simulink model "autopilot3d"  (R2017a)
settings: Solver=VariableStepAuto  StartTime=0.0  StopTime=300  RelTol=1e-3
values from neighbouring files (symbols this model uses):
  A = [-0.322     0.052   0.028   -1.12   0.002 ... (first row only)    [run_task_3e.m]
  A_kal = A(1:4, 1:4)    [run_task_3e.m]
  B = [0; 0; 0; 0; 10]    [run_task_3e.m]
  B_kal = A(1:4,5)    [run_task_3e.m]
  C = [0 0 0 1 0 ... (first row only)    [run_task_3e.m]
  C_kal = [0 0 0 1 ... (first row only)    [run_task_3e.m]
  d = 2*deg2rad    (= 0.0349065850399)    [run_task_3e.m]
  D = zeros(4, 1)    [run_task_3e.m]
  g = 9.81    [run_task_3e.m]
  k_d_phi = (2*zeta_phi*w_n_phi-a_1)/a_2    [run_task_3e.m]
  k_i_x = 0.195    [run_task_3e.m]
  k_p_phi = -5/3    (= -1.66666666667)    [run_task_3e.m]
  k_p_x = 2*zeta_X*w_n_x*V_g/g    [run_task_3e.m]
  large_step = 30    [run_task_3e.m]
  P = [1 0 0 0 ... (first row only)    [run_task_3e.m]
  Q = [1 0 0 0 ... (first row only)    [run_task_3e.m]
  R = [r_noise_var 0 0 ... (first row only)    [run_task_3e.m]
  step_size = 0.001    [run_task_3e.m]
  V_g = 637/3.6    (= 176.944444444)    [run_task_3e.m]
  x_hat = x_hat_init    [run_task_3e.m]
libraries: simulink_extras x3
settings Model: Creator=rokru  LastModifiedBy=emilal

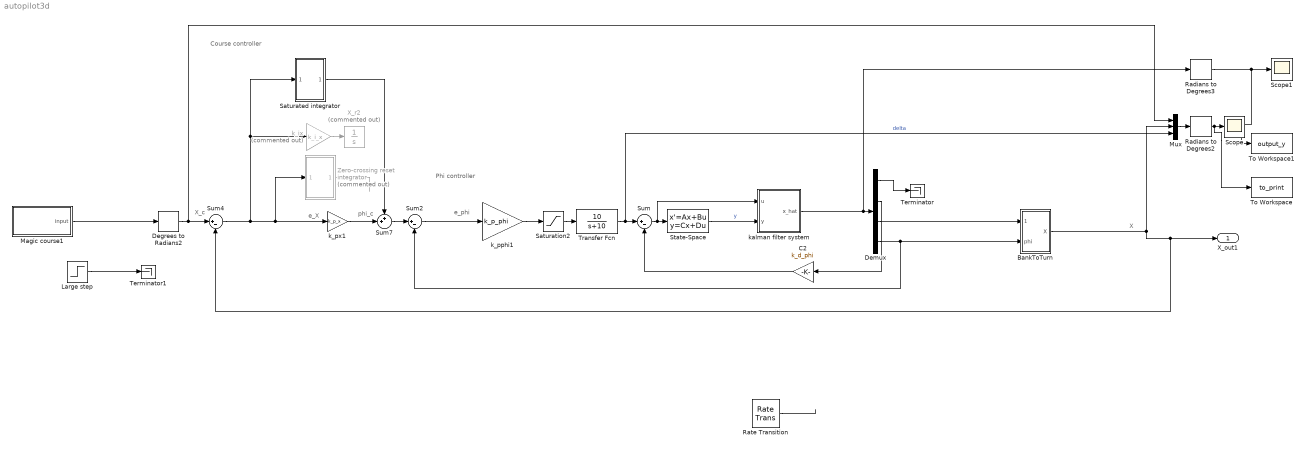
== system autopilot3d ==
  note: X
  note: X_c
  note: phi_c
  note: Course controller
  note: e_X
  note: Phi controller
  note: e_phi
  BankToTurn : Subsystem
  C2 : Gain  Gain=k_d_phi
  Degrees to Radians2 : simulink_extras/Transformations/Degrees to Radians
  Demux : Demux
  Large step : Step  Time=50  After=large_step  SampleTime=0
  Magic course1 : Subsystem
  Mux : Mux  Inputs=3
  Radians to Degrees2 : simulink_extras/Transformations/Radians to Degrees
  Radians to Degrees3 : simulink_extras/Transformations/Radians to Degrees
  Rate Transition : RateTransition
  Saturated integrator : Subsystem
  Saturation2 : Saturate  UpperLimit=25*deg2rad  LowerLimit=-25*deg2rad
  Scope : Scope
  Scope1 : Scope
  State-Space : StateSpace  A=A  B=B  C=C  D=D  X0=0
  Sum : Sum  Inputs=|+-
  Sum2 : Sum  Inputs=|+-
  Sum4 : Sum  Inputs=|+-
  Sum7 : Sum  Inputs=++|
  Terminator : Terminator
  Terminator1 : Terminator
  To Workspace : ToWorkspace  VariableName=to_print  SaveFormat=Timeseries  SampleTime=-1
  To Workspace1 : ToWorkspace  VariableName=output_y  SaveFormat=Timeseries  SampleTime=-1
  Transfer Fcn : TransferFcn  Numerator=[10]  Denominator=[1 10]
  X_r2 : Integrator  Commented=on
  "Zero-crossing reset integrator " : Subsystem  Commented=on
  k_ix : Gain  Commented=on  Gain=k_i_x
  k_pphi1 : Gain  Gain=k_p_phi
  k_px1 : Gain  Gain=k_p_x
  kalman filter system : Subsystem
  X_out1 : Outport
  wires:
  k_px1/1 -> Sum7/2
  Sum4/1 -> Saturated integrator/1(In1), k_ix/1, "Zero-crossing reset integrator "/1(In1), k_px1/1
  C2/1 -> Sum/2
  Saturation2/1 -> Transfer Fcn/1
  Mux/1 -> Radians to Degrees2/1
  Demux/2 -> C2/1
  Demux/4 -> Sum2/2, BankToTurn/2(phi)
  Sum/1 -> kalman filter system/1(u), State-Space/1
  k_pphi1/1 -> Saturation2/1
  Sum7/1 -> Sum2/1
  Sum2/1 -> k_pphi1/1
  Magic course1/1(input) -> Degrees to Radians2/1
  Transfer Fcn/1 -> Sum/1, Mux/3  "delta"
  Degrees to Radians2/1 -> Mux/1, Sum4/1
  Radians to Degrees3/1 -> To Workspace1/1, Scope1/1
  Radians to Degrees2/1 -> To Workspace/1, Scope/1
  Demux/1 -> Terminator/1
  Large step/1 -> Terminator1/1
  "Zero-crossing reset integrator "/1(Out1) -> ?
  k_ix/1 -> X_r2/1
  Saturated integrator/1(Out1) -> Sum7/1
  BankToTurn/1(X) -> Sum4/2, X_out1/1, Mux/2
  Demux/3 -> BankToTurn/1(sideslip)
  kalman filter system/1(x_hat) -> Radians to Degrees3/1, Demux/1
  State-Space/1 -> kalman filter system/2(y)  "y"
  Rate Transition/1 -> ?

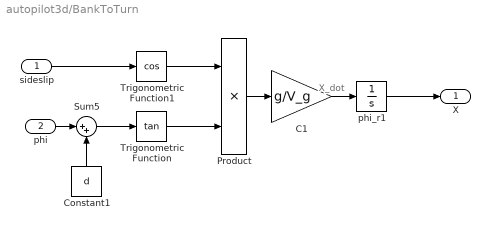
== system autopilot3d/BankToTurn ==
  note: X_dot
  sideslip : Inport
  phi : Inport  Port=2
  C1 : Gain  Gain=g/V_g
  Constant1 : Constant  Value=d
  Product : Product
  Sum5 : Sum  Inputs=|++
  Trigonometric Function : Trigonometry  Operator=tan
  Trigonometric Function1 : Trigonometry  Operator=cos
  phi_r1 : Integrator
  X : Outport
  wires:
  Trigonometric Function/1 -> Product/2
  C1/1 -> phi_r1/1
  Product/1 -> C1/1
  sideslip/1 -> Trigonometric Function1/1
  Trigonometric Function1/1 -> Product/1
  Constant1/1 -> Sum5/2
  Sum5/1 -> Trigonometric Function/1
  phi_r1/1 -> X/1
  phi/1 -> Sum5/1

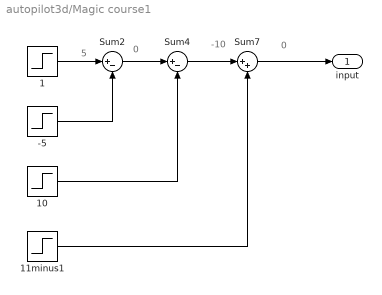
== system autopilot3d/Magic course1 ==
  note: 0
  note: -10
  note: 0
  note: 5
  -5 : Step  Time=100  After=5  SampleTime=0
  1 : Step  Time=10  After=5  SampleTime=0
  10 : Step  Time=150  After=10  SampleTime=0
  11minus1 : Step  Time=200  After=10  SampleTime=0
  Sum2 : Sum  Inputs=|+-
  Sum4 : Sum  Inputs=|+-
  Sum7 : Sum  Inputs=|++
  input : Outport
  wires:
  10/1 -> Sum4/2
  11minus1/1 -> Sum7/2
  -5/1 -> Sum2/2
  Sum7/1 -> input/1
  1/1 -> Sum2/1
  Sum4/1 -> Sum7/1
  Sum2/1 -> Sum4/1

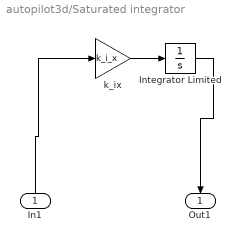
== system autopilot3d/Saturated integrator ==
  In1 : Inport
  Integrator Limited : Integrator  LimitOutput=on  UpperSaturationLimit=0.06  LowerSaturationLimit=-0.06
  k_ix : Gain  Gain=k_i_x
  Out1 : Outport
  wires:
  k_ix/1 -> Integrator Limited/1
  Integrator Limited/1 -> Out1/1
  In1/1 -> k_ix/1

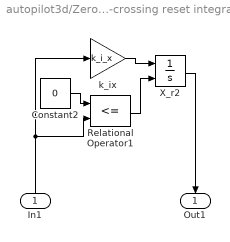
== system autopilot3d/Zero-crossing reset integrator  ==
  In1 : Inport
  Constant2 : Constant  Value=0
  Relational Operator1 : RelationalOperator  Operator=<=  OutDataTypeStr=boolean  RndMeth=Simplest
  X_r2 : Integrator  ExternalReset=level
  k_ix : Gain  Gain=k_i_x
  Out1 : Outport
  wires:
  Constant2/1 -> Relational Operator1/1
  Relational Operator1/1 -> X_r2/2
  k_ix/1 -> X_r2/1
  X_r2/1 -> Out1/1
  In1/1 -> Relational Operator1/2, k_ix/1

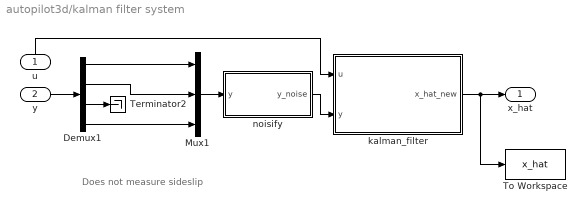
== system autopilot3d/kalman filter system ==
  note: Does not measure sideslip
  u : Inport
  y : Inport  Port=2
  Demux1 : Demux
  Mux1 : Mux  Inputs=3
  Terminator2 : Terminator
  To Workspace : ToWorkspace  VariableName=x_hat  SaveFormat=Timeseries  SampleTime=-1
  kalman_filter : MATLAB Function  TreatAsAtomicUnit=on
  noisify : MATLAB Function  TreatAsAtomicUnit=on
  x_hat : Outport
  wires:
  Demux1/1 -> Mux1/1
  Demux1/3 -> Terminator2/1
  Mux1/1 -> noisify/1(y)
  Demux1/4 -> Mux1/3
  y/1 -> Demux1/1
  Demux1/2 -> Mux1/2
  u/1 -> kalman_filter/1(u)
  kalman_filter/1(x_hat_new) -> To Workspace/1, x_hat/1
  noisify/1(y_noise) -> kalman_filter/2(y)

== matlab function autopilot3d/kalman filter system/kalman_filter ==
  data: u input; y input; x_hat_new output; P parameter; A_kal parameter; B_kal parameter; C_kal parameter; E parameter; R parameter; Q parameter; step_size parameter; x_hat parameter
function x_hat_new   = kalman_filter(u, y, P, A_kal, B_kal, C_kal, E, R, Q, step_size, x_hat)


%from p. 297 in Fossen
K = P*C_kal' / (R);
x_hat_dot = A_kal*x_hat + B_kal*u + K*(y - C_kal*x_hat);
P_dot = A_kal*P + P*A_kal'  + E*Q*E' - (P*C_kal'/R)*C_kal*P;

%Updating x_hat and P. Too trivial way?
P = P + P_dot * step_size;
x_hat_new = x_hat + x_hat_dot * step_size;
end

== matlab function autopilot3d/kalman filter system/noisify ==
  data: y input; y_noise output
function y_noise   = noisify(y)

r_noise_var = 0.2; % (deg/s)^2 
p_noise_var = 0.5; % (deg/s)^2
phi_noise_var = 2; % (deg)^2

vars = [r_noise_var; p_noise_var; phi_noise_var];

y_noise = y + randn(1,3)* vars;

end
